simulink model "autosar_tpc_system"  (R2022b)
settings: Solver=FixedStepAuto  StartTime=0  StopTime=1.1  FixedStep=.005  RelTol=1e-3  EnableMultiTasking=on
model workspace (MAT data in the model file):
  J = 0.226199211484
  Kt = 174.53
  Ts_verif = Simulink.Parameter
  Ts_verif.Value = 0.001
  Ts_verif.DataType = 'auto'
  Ts_verif.Complexity = 'real'
  Ts_verif.Dimensions = [1 1]
  angle_init = 15
  angle_open = 85
  c = 8.89069171842
  fall_end_angle = Simulink.Parameter
  fall_end_angle.Value = 0.1
  fall_end_angle.DataType = 'auto'
  fall_end_angle.Complexity = 'real'
  fall_end_angle.Dimensions = [1 1]
  fall_start_angle = Simulink.Parameter
  fall_start_angle.Value = 0.9
  fall_start_angle.DataType = 'auto'
  fall_start_angle.Complexity = 'real'
  fall_start_angle.Dimensions = [1 1]
  input_delay = 0.00986306560803
  k = 19.1559540807
  rise_end_angle = Simulink.Parameter
  rise_end_angle.Value = 0.9
  rise_end_angle.DataType = 'auto'
  rise_end_angle.Complexity = 'real'
  rise_end_angle.Dimensions = [1 1]
  rise_start_angle = Simulink.Parameter
  rise_start_angle.Value = 0.1
  rise_start_angle.DataType = 'auto'
  rise_start_angle.Complexity = 'real'
  rise_start_angle.Dimensions = [1 1]
  vv_fall_time_max = Simulink.Parameter
  vv_fall_time_max.Value = 0.3
  vv_fall_time_max.DataType = 'auto'
  vv_fall_time_max.Complexity = 'real'
  vv_fall_time_max.Dimensions = [1 1]
  vv_fall_time_min = Simulink.Parameter
  vv_fall_time_min.Value = 0.001
  vv_fall_time_min.DataType = 'auto'
  vv_fall_time_min.Complexity = 'real'
  vv_fall_time_min.Dimensions = [1 1]
  vv_rise_time_max = Simulink.Parameter
  vv_rise_time_max.Value = 0.1
  vv_rise_time_max.DataType = 'auto'
  vv_rise_time_max.Complexity = 'real'
  vv_rise_time_max.Dimensions = [1 1]
  vv_rise_time_min = Simulink.Parameter
  vv_rise_time_min.Value = 0.001
  vv_rise_time_min.DataType = 'auto'
  vv_rise_time_min.Complexity = 'real'
  vv_rise_time_min.Dimensions = [1 1]
libraries: SignalEditorBlockLib x1
settings Model: Creator=The MathWorks, Inc.  LastModifiedBy=The MathWorks, Inc.
settings SolverCC: AlgebraicLoopSolver=TrustRegion  AutoInsertRateTranBlk=on  InsertRTBMode=Never (minimum delay)
settings DataIOCC: SaveFormat=Array  SaveOutput=off  SignalLogging=off  DSMLogging=off  SaveTime=off  ReturnWorkspaceOutputs=off  SignalLoggingName=DataLog
settings OptimizationCC: BooleanDataType=off  DefaultParameterBehavior=Inlined  InlineInvariantSignals=on  ExpressionDepthLimit=2147483647  InitFltsAndDblsToZero=on  NoFixptDivByZeroProtection=on  EfficientFloat2IntCast=on  LifeSpan=1  BufferReusableBoundary=off  EfficientTunableParamExpr=on
settings DebuggingCC: SaveWithParameterizedLinksMsg=none  MultiTaskDSMMsg=none  MultiTaskRateTransMsg=warning  IntegerOverflowMsg=none  FcnCallInpInsideContextMsg=warning  UnconnectedInputMsg=warning  UnconnectedOutputMsg=warning  UnconnectedLineMsg=warning  BusObjectLabelMismatch=none  StateNameClashWarn=warning  SFUnexpectedBacktrackingDiag=warning  SFNoUnconditionalDefaultTransitionDiag=warning  SFExecutionAtInitializationDiag=none  SFMachineParentedDataDiag=warning  ArithmeticOperatorsInVariantConditions=warning
settings HardwareCC: ProdBitPerPointer=32  ProdBitPerSizeT=32  ProdBitPerPtrDiffT=32  ProdLargestAtomicFloat=None  ProdIntDivRoundTo=Undefined  ProdEndianess=Unspecified  ProdWordSize=32  ProdHWDeviceType=32-bit Generic
settings ModelReferenceCC: EnableRefExpFcnMdlSchedulingChecks=on  PropagateSignalLabelsOutOfModel=off
settings SFSimCC: SimUseLocalCustomCode=off  SimParseCustomCode=off  MATLABDynamicMemAlloc=off
settings RTWCC: Description=Real-Time Workshop Embedded Coder (no auto configuration)  SystemTargetFile=ert.tlc  TemplateMakefile=ert_default_tmf  GenerateReport=on  RTWUseLocalCustomCode=off  IncludeHyperlinkInReport=on  LaunchReport=on
settings CodeAppCC: IgnoreCustomStorageClasses=off  SimulinkDataObjDesc=on  CustomSymbolStrType=$N$R$M  StateflowObjectComments=on  InternalIdentifier=Classic  ReqsInCode=on
settings ERTTargetCC: TargetFcnLib=ansi_tfl_tmw.mat  UtilityFuncGeneration=Shared location  MultiwordLength=2048  GenerateSampleERTMain=on  IncludeMdlTerminateFcn=off  SuppressErrorStatus=on  SupportAbsoluteTime=off  SupportNonFinite=off  SupportComplex=off  InlinedParameterPlacement=NonHierarchical  ERTSrcFileBannerTemplate=eng_ctrl_code_template.cgt  ERTCustomFileTemplate=example_file_process.tlc  ConvertIfToSwitch=off  SuppressUnreachableDefaultCases=off
settings ConfigComp: CovMetricSettings=dw  CovSaveCumulativeToWorkspaceVar=on  CovSaveSingleToWorkspaceVar=on  CovExternalEMLEnable=off
settings SimscapeCC: SimscapeNormalizeSystem=off

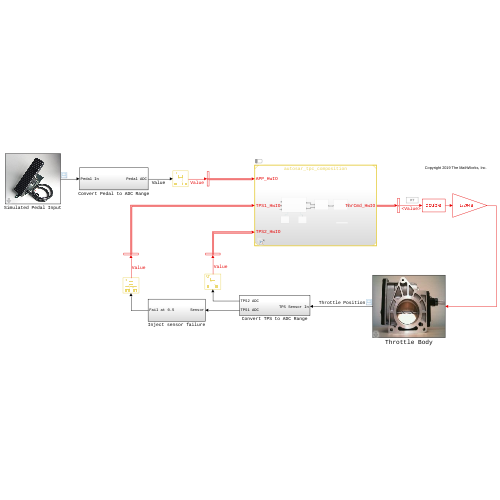
[thumbnail: Simulink's stored preview of the top-level diagram]
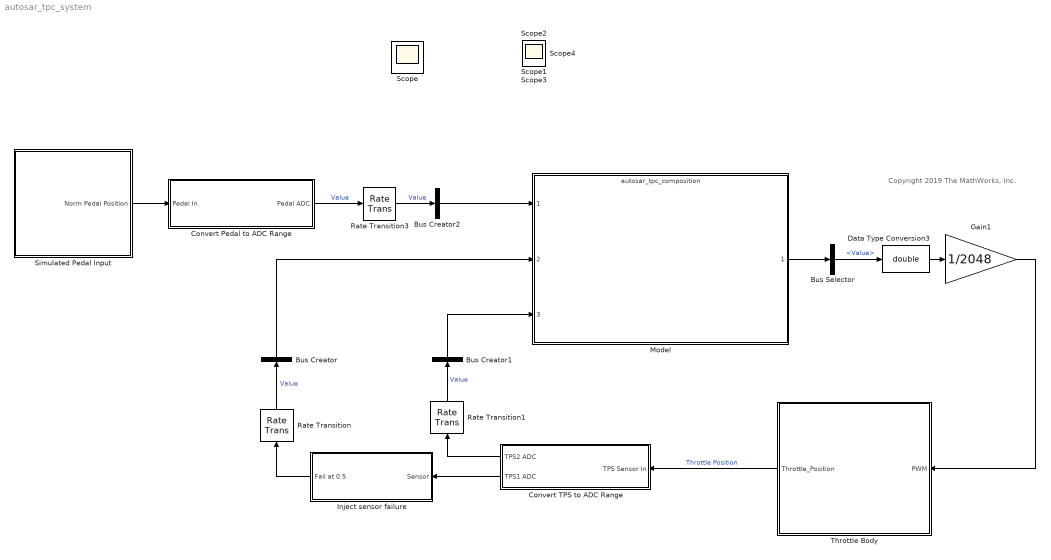
== system autosar_tpc_system ==
  note: Copyright 2019 The MathWorks, Inc.
  Bus Creator : BusCreator  Inputs=1
  Bus Creator1 : BusCreator  Inputs=1
  Bus Creator2 : BusCreator  Inputs=1
  Bus Selector : BusSelector  OutputSignals=Value
  Convert Pedal to ADC Range : Subsystem
  Convert TPS to ADC Range : Subsystem
  Data Type Conversion3 : DataTypeConversion  OutDataTypeStr=double  SaturateOnIntegerOverflow=off  RndMeth=Floor
  Gain1 : Gain  Gain=1/2048
  Inject sensor failure : Subsystem
  Model : ModelReference  ModelNameDialog=autosar_tpc_composition.slx  SimulationMode=Normal  ScheduleRates=on  ScheduleRatesWith=Schedule Editor  HasExplicitPartitions=on  ModelReferenceVersion=6.1
  Rate Transition : RateTransition  Deterministic=off  OutPortSampleTime=.005
  Rate Transition1 : RateTransition  Deterministic=off  OutPortSampleTime=.005
  Rate Transition3 : RateTransition  Deterministic=off  OutPortSampleTime=.005
  Simulated Pedal Input : Subsystem  mask{groupIndex=60% Pulse}
      mask prompts: groupIndex "Select Signal Group"
      mask help:
      | To use this block in a Simulink model, add the following code to the model
      | InitFcn callback:
      | groupIndex = get_param([gcs,'/Simulated Pedal Input'], 'MaskWSVariables');
      | signalbuilder([gcs,'/Simulated Pedal Input/Test Signals'], 'activegroup', groupIndex.Value);
      mask TypeOptions groupIndex: WOT Step | 60% Pulse | Sinusoidal Pulsetrain
      mask Callback groupIndex:
      | sourceBlk = [gcb '/Test Signals'];
      |     selectedScenario = get_param(gcb,'groupIndex');
      |     switch selectedScenario
      |         case 'WOT Step'
      |             selectedScenario = 'WOT_Step';
      |         case '60% Pulse'
      |             selectedScenario = 'Test_Case_60_Pulse';
      |         case 'Sinusoidal Pulsetrain'
      |             selectedScenario = 'Pulse';
      |     end
      |     set_param(sourceBlk,'ActiveScenario',selectedScenario);
      mask Display: image('pedal.jpg')
  Throttle Body : Subsystem  mask{units=normalized, input_delay=input_delay, J=J, c=c, k=k, close_angle=angle_init, open_angle=angle_open}
      mask prompts: input_delay "Input Delay:"; J "Inertia:"; c "Damping:"; k "Stiffness:"; close_angle "Resting Angle:"; open_angle "Open Angle:"
      mask TypeOptions units: rads | degrees | normalized
      mask Display: image('throttle.jpg')
  Scope{,1..4} (5 alike) : Scope
  wires:
  Gain1/1 -> Throttle Body/1(PWM)
  Data Type Conversion3/1 -> Gain1/1
  Throttle Body/1(Throttle_Position) -> Convert TPS to ADC Range/1(TPS Sensor In)  "Throttle Position"
  Simulated Pedal Input/1(Norm Pedal Position) -> Convert Pedal to ADC Range/1(Pedal In)
  Convert TPS to ADC Range/1(TPS2 ADC) -> Rate Transition1/1
  Rate Transition/1 -> Bus Creator/1  "Value"
  Bus Creator/1 -> Model/2
  Rate Transition1/1 -> Bus Creator1/1  "Value"
  Bus Creator1/1 -> Model/3
  Convert Pedal to ADC Range/1(Pedal ADC) -> Rate Transition3/1  "Value"
  Bus Creator2/1 -> Model/1
  Model/1 -> Bus Selector/1
  Bus Selector/1 -> Data Type Conversion3/1  "<Value>"
  Rate Transition3/1 -> Bus Creator2/1  "Value"
  Convert TPS to ADC Range/2(TPS1 ADC) -> Inject sensor failure/1(Sensor)
  Inject sensor failure/1(Fail at 0.5) -> Rate Transition/1

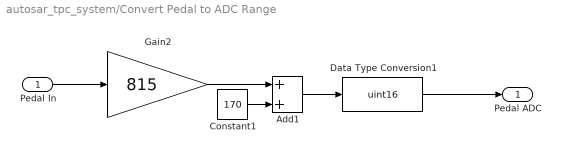
== system autosar_tpc_system/Convert Pedal to ADC Range ==
  Pedal In : Inport
  Add1 : Sum
  Constant1 : Constant  Value=170
  Data Type Conversion1 : DataTypeConversion  OutDataTypeStr=uint16  SaturateOnIntegerOverflow=off  RndMeth=Floor
  Gain2 : Gain  Gain=815
  Pedal ADC : Outport  VectorParamsAs1DForOutWhenUnconnected=off
  wires:
  Gain2/1 -> Add1/1
  Constant1/1 -> Add1/2
  Data Type Conversion1/1 -> Pedal ADC/1
  Add1/1 -> Data Type Conversion1/1
  Pedal In/1 -> Gain2/1

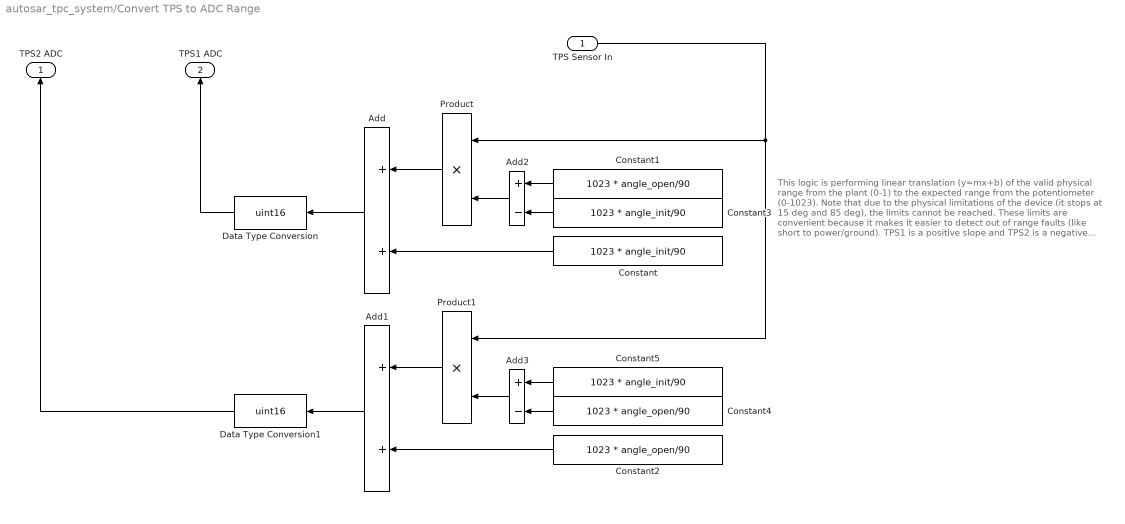
== system autosar_tpc_system/Convert TPS to ADC Range ==
  note: This logic is performing linear translation (y=mx+b) of the valid physical range from the plant (0-1) to the expected range from the potentiometer (0-1023).
      |
      | Note that due to the physical limitations of the device (it stops at 15 deg and 85 deg), the limits cannot be reached.
      |
      | These limits are convenient because it makes it easier to detect out of range faults (like short to power/ground).
      |
      | TPS1 is a positive slope and TPS2 is a negative slope.  This is common in these devices so cross checking between the two sensors can be performed.
  TPS Sensor In : Inport
  Add : Sum
  Add1 : Sum
  Add2 : Sum  Inputs=+-
  Add3 : Sum  Inputs=+-
  Constant : Constant  Value=1023 * angle_init/90
  Constant1 : Constant  Value=1023 * angle_open/90
  Constant2 : Constant  Value=1023 * angle_open/90
  Constant3 : Constant  Value=1023 * angle_init/90
  Constant4 : Constant  Value=1023 * angle_open/90
  Constant5 : Constant  Value=1023 * angle_init/90
  Data Type Conversion : DataTypeConversion  OutDataTypeStr=uint16  SaturateOnIntegerOverflow=off  RndMeth=Floor
  Data Type Conversion1 : DataTypeConversion  OutDataTypeStr=uint16  SaturateOnIntegerOverflow=off  RndMeth=Floor
  Product : Product
  Product1 : Product
  TPS2 ADC : Outport  VectorParamsAs1DForOutWhenUnconnected=off
  TPS1 ADC : Outport  Port=2  VectorParamsAs1DForOutWhenUnconnected=off
  wires:
  Product/1 -> Add/1
  Constant/1 -> Add/2
  Add/1 -> Data Type Conversion/1
  Data Type Conversion/1 -> TPS1 ADC/1
  Add1/1 -> Data Type Conversion1/1
  Add2/1 -> Product/2
  Constant1/1 -> Add2/1
  Constant3/1 -> Add2/2
  Constant4/1 -> Add3/2
  Constant5/1 -> Add3/1
  Add3/1 -> Product1/2
  Constant2/1 -> Add1/2
  Product1/1 -> Add1/1
  Data Type Conversion1/1 -> TPS2 ADC/1
  TPS Sensor In/1 -> Product1/1, Product/1

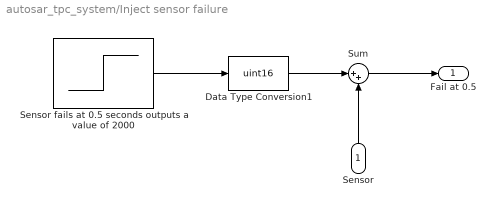
== system autosar_tpc_system/Inject sensor failure ==
  Sensor : Inport
  Data Type Conversion1 : DataTypeConversion  OutDataTypeStr=uint16  SaturateOnIntegerOverflow=off  RndMeth=Floor
  Sensor fails at 0.5 seconds outputs a value of 2000 : Step  Time=0.5  After=2000  SampleTime=0
  Sum : Sum  Inputs=|++
  Fail at 0.5 : Outport
  wires:
  Sensor fails at 0.5 seconds outputs a value of 2000/1 -> Data Type Conversion1/1
  Sum/1 -> Fail at 0.5/1
  Data Type Conversion1/1 -> Sum/1
  Sensor/1 -> Sum/2

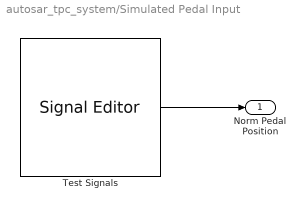
== system autosar_tpc_system/Simulated Pedal Input ==
  Test Signals : SignalEditorBlockLib/Signal Editor  FileName=PedalInput.mat  ActiveScenario=Test_Case_60_Pulse  ActiveSignal=a  IsBus=off  OutputBusObjectStr=Bus: BusObject  SampleTime=0  ZeroCross=off  OutputAfterFinalValue=Extrapolation  Unit=inherit  PreserveSignalName=on
  Norm Pedal Position : Outport  VectorParamsAs1DForOutWhenUnconnected=off
  wires:
  Test Signals/1 -> Norm Pedal Position/1

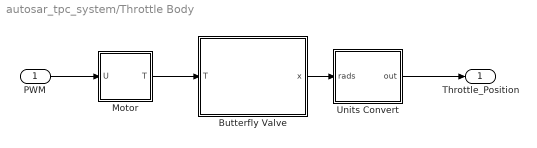
== system autosar_tpc_system/Throttle Body ==
  PWM : Inport
  Butterfly Valve : Subsystem  mask{var_J=J, var_D=c, var_K=k, angle_init=angle_init, angle_open=angle_open}
      mask prompts: var_J "Inertia:"; var_D "Damping:"; var_K "Stiffness:"; angle_init "Resting Angle:"; angle_open "Open Angle:"
  Motor : Subsystem
  Units Convert : Subsystem
  Throttle_Position : Outport  VectorParamsAs1DForOutWhenUnconnected=off
  wires:
  PWM/1 -> Motor/1(U)
  Motor/1(T) -> Butterfly Valve/1(T)
  Units Convert/1(out) -> Throttle_Position/1
  Butterfly Valve/1(x) -> Units Convert/1(rads)

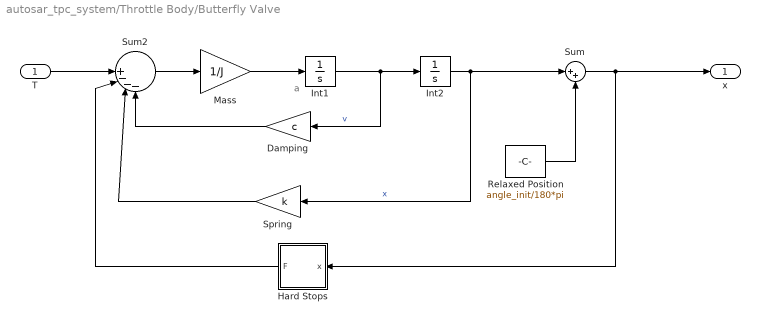
== system autosar_tpc_system/Throttle Body/Butterfly Valve ==
  note: a
  T : Inport
  Damping : Gain  Gain=c  SaturateOnIntegerOverflow=on  OutDataTypeStr=Inherit: Same as input  ParamDataTypeStr=Inherit: Same as input
  Hard Stops : Subsystem  mask{H=angle_open/180*pi, K=2.86e5, L=angle_init/180*pi}
      mask prompts: H "Upper Limit:"; K "Stiffness:"; L "Lower Limit:"
  Int1 : Integrator
  Int2 : Integrator
  Mass : Gain  Gain=1/J  SaturateOnIntegerOverflow=on  OutDataTypeStr=Inherit: Same as input  ParamDataTypeStr=Inherit: Same as input
  Relaxed Position : Constant  Value=angle_init/180*pi
  Spring : Gain  Gain=k  SaturateOnIntegerOverflow=on  OutDataTypeStr=Inherit: Same as input  ParamDataTypeStr=Inherit: Same as input
  Sum : Sum  Inputs=|++  InputSameDT=on  SaturateOnIntegerOverflow=on  OutDataTypeStr=Inherit: Same as first input
  Sum2 : Sum  Inputs=|||+---  InputSameDT=on  SaturateOnIntegerOverflow=on  OutDataTypeStr=Inherit: Same as first input
  x : Outport  VectorParamsAs1DForOutWhenUnconnected=off
  wires:
  Hard Stops/1(F) -> Sum2/2
  Spring/1 -> Sum2/3
  Int2/1 -> Spring/1, Sum/1  "x"
  Relaxed Position/1 -> Sum/2
  Sum2/1 -> Mass/1
  T/1 -> Sum2/1
  Mass/1 -> Int1/1
  Int1/1 -> Damping/1, Int2/1  "v"
  Damping/1 -> Sum2/4
  Sum/1 -> x/1, Hard Stops/1(x)

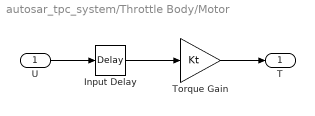
== system autosar_tpc_system/Throttle Body/Motor ==
  U : Inport
  Input Delay : TransportDelay  DelayTime=input_delay
  Torque Gain : Gain  Gain=Kt  SaturateOnIntegerOverflow=on  OutDataTypeStr=Inherit: Same as input  ParamDataTypeStr=Inherit: Same as input
  T : Outport  VectorParamsAs1DForOutWhenUnconnected=off
  wires:
  U/1 -> Input Delay/1
  Torque Gain/1 -> T/1
  Input Delay/1 -> Torque Gain/1

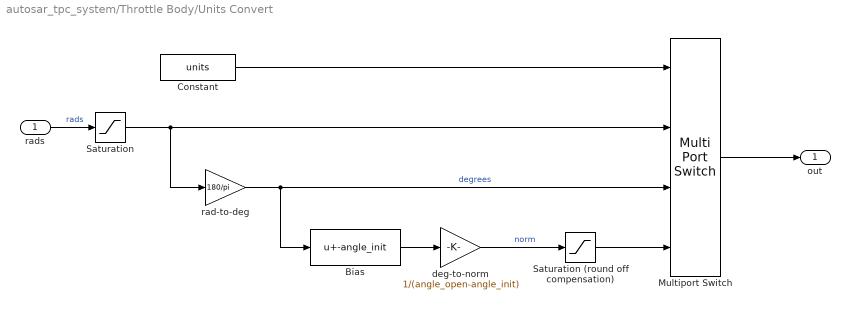
== system autosar_tpc_system/Throttle Body/Units Convert ==
  rads : Inport
  Bias : Bias  Bias=-angle_init  SaturateOnIntegerOverflow=off
  Constant : Constant  Value=units
  Multiport Switch : MultiPortSwitch  SaturateOnIntegerOverflow=off  InputSameDT=off
  Saturation : Saturate  UpperLimit=pi/2  LowerLimit=0.0
  Saturation (round off compensation) : Saturate  UpperLimit=1.0  LowerLimit=0.0
  deg-to-norm : Gain  Gain=1/(angle_open-angle_init)
      settings: AttributesFormatString=%<Gain>
  rad-to-deg : Gain  Gain=180/pi
  out : Outport  VectorParamsAs1DForOutWhenUnconnected=off
  wires:
  Saturation/1 -> rad-to-deg/1, Multiport Switch/2
  Saturation (round off compensation)/1 -> Multiport Switch/4
  Bias/1 -> deg-to-norm/1
  deg-to-norm/1 -> Saturation (round off compensation)/1  "norm"
  Constant/1 -> Multiport Switch/1
  Multiport Switch/1 -> out/1
  rads/1 -> Saturation/1  "rads"
  rad-to-deg/1 -> Multiport Switch/3, Bias/1  "degrees"

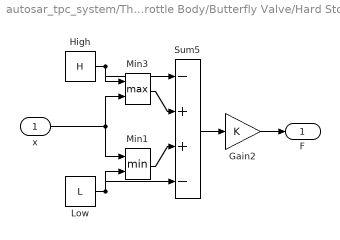
== system autosar_tpc_system/Throttle Body/Butterfly Valve/Hard Stops ==
  x : Inport
  Gain2 : Gain  Gain=K  SaturateOnIntegerOverflow=on  OutDataTypeStr=Inherit: Same as input  ParamDataTypeStr=Inherit: Same as input
  High : Constant  Value=H
  Low : Constant  Value=L
  Min1 : MinMax  Inputs=2  InputSameDT=on  SaturateOnIntegerOverflow=on
  Min3 : MinMax  Function=max  Inputs=2  InputSameDT=on  SaturateOnIntegerOverflow=on
  Sum5 : Sum  Inputs=-+||+-  InputSameDT=on  SaturateOnIntegerOverflow=on  OutDataTypeStr=Inherit: Same as first input
  F : Outport  VectorParamsAs1DForOutWhenUnconnected=off
  wires:
  Gain2/1 -> F/1
  x/1 -> Min1/1, Min3/2
  Sum5/1 -> Gain2/1
  Low/1 -> Min1/2, Sum5/4
  High/1 -> Sum5/1, Min3/1
  Min3/1 -> Sum5/2
  Min1/1 -> Sum5/3
